simulink model "benchmark_ivan_PIANN"  (R2024b)
settings: Solver=FixedStepAuto  StartTime=0.0  StopTime=14  FixedStep=0.0001  RelTol=1e-5  AbsTol=1e-8  EnableMultiTasking=on
values from neighbouring files (symbols this model uses):
  b1 = csvread('./DAE_ANN/ANN/Biases/30_04_21/lstm_ann_pi_standard_fix_noSo4_rnn_1__100_16_b_3.csv')    [init_PI_ann.m]    (also in init_PI_ann_hier.m = csvread('./DAE_ANN/ANN/Biases/12_05_21/lstm_ann_pi_standard_; init_PI_ann_hier_v2.m = csvread('./DAE_ANN/ANN/Biases/12_05_21/lstm_ann_pi_standard_; init_PI_ann_lab.m = csvread('./DAE_ANN/ANN/Biases/12_05_21/lstm_ann_pi_standard_)
  b2 = csvread('./DAE_ANN/ANN/Biases/30_04_21/lstm_ann_pi_standard_fix_noSo4_rnn_1__100_16_b_3.csv')    [init_PI_ann.m]    (also in init_PI_ann_hier.m = csvread('./DAE_ANN/ANN/Biases/12_05_21/lstm_ann_pi_standard_; init_PI_ann_hier_v2.m = csvread('./DAE_ANN/ANN/Biases/12_05_21/lstm_ann_pi_standard_; init_PI_ann_lab.m = csvread('./DAE_ANN/ANN/Biases/12_05_21/lstm_ann_pi_standard_)
  b_last = csvread('./DAE_ANN/ANN/Biases/12_05_21/lstm_ann_pi_standard_fix_noSo4_last__100_1_b_2.csv')'    [init_PI_ann_hier.m]    (also in init_PI_ann_hier_v2.m; init_PI_ann_lab.m)
  b_out = csvread('./DAE_ANN/ANN/Biases/30_04_21/lstm_ann_pi_standard_fix_noSo4_final__100_16_b_3.csv')    [init_PI_ann.m]    (also in init_PI_ann_hier.m = csvread('./DAE_ANN/ANN/Biases/12_05_21/lstm_ann_pi_standard_; init_PI_ann_hier_v2.m = csvread('./DAE_ANN/ANN/Biases/12_05_21/lstm_ann_pi_standard_; init_PI_ann_lab.m = csvread('./DAE_ANN/ANN/Biases/12_05_21/lstm_ann_pi_standard_)
  ic_sw_Kla = 145*ones(n_sw,1)    [init_PI_ann.m]    (also in init_PI_ann_hier.m; init_PI_ann_hier_v2.m; init_PI_ann_lab.m)
  ic_sw_Snh4 = 6*ones(n_sw,1)    [init_PI_ann.m]    (also in init_PI_ann_hier.m; init_PI_ann_hier_v2.m; init_PI_ann_lab.m)
  ic_sw_Sno4 = 8*ones(n_sw,1)    [init_PI_ann.m]    (also in init_PI_ann_hier.m; init_PI_ann_hier_v2.m; init_PI_ann_lab.m)
  ic_sw_So4 = 3*ones(n_sw,1)    [init_PI_ann.m]    (also in init_PI_ann_hier.m; init_PI_ann_hier_v2.m; init_PI_ann_lab.m)
  ic_sw_So5 = 2*ones(n_sw,1)    [init_PI_ann.m]    (also in init_PI_ann_hier.m; init_PI_ann_hier_v2.m; init_PI_ann_lab.m)
  KLa5_max = 360    [sensorinit.m]
  max_Q4 = 100000    [sensorinit.m]
  max_SNH4 = 20    [sensorinit.m]
  max_SNO2 = 20    [sensorinit.m]
  max_SNO4 = 20    [sensorinit.m]
  max_SO4 = 10    [sensorinit.m]
  max_SO5 = 10    [sensorinit.m]    (also in setup_Prac5.m = 5)
  max_TSS4 = 10000    [sensorinit.m]
  mean_scaler_dir = csvread('./DAE_ANN/ANN/Scalers/30_04_21_lstm_ann_pi_standard_fix_noSo4/mean_scaler_lstm_ann_pi_standard_fix_noSo4.csv')    [init_PI_ann.m]    (also in init_PI_ann_hier.m = csvread('./DAE_ANN/ANN/Scalers/12_05_21_lstm_ann_pi_standard; init_PI_ann_hier_v2.m = csvread('./DAE_ANN/ANN/Scalers/12_05_21_lstm_ann_pi_standard; setup_Prac5.m = [(Q/k)^2, 1.9756, 0.0000, 0]')
  mean_scaler_dir_out = csvread('./DAE_ANN/ANN/Scalers/30_04_21_lstm_ann_pi_standard_fix_noSo4/mean_scaler_lstm_ann_pi_standard_fix_noSo4_out.csv')    [init_PI_ann.m]    (also in init_PI_ann_hier.m = csvread('./DAE_ANN/ANN/Scalers/12_05_21_lstm_ann_pi_standard; init_PI_ann_hier_v2.m = csvread('./DAE_ANN/ANN/Scalers/12_05_21_lstm_ann_pi_standard; setup_Prac5.m = 0)
  min_Q4 = 0    [sensorinit.m]
  min_SNH4 = 0    [sensorinit.m]
  min_SNO2 = 0    [sensorinit.m]
  min_SNO4 = 0    [sensorinit.m]
  min_SO5 = 0    [sensorinit.m]
  min_TSS4 = 0    [sensorinit.m]
  n_layers = 1    [init_PI_ann.m]    (also in init_PI_ann_hier.m; init_PI_ann_hier_v2.m; init_PI_ann_lab.m)
  n_sw = 16    [init_PI_ann.m]    (also in init_PI_ann_hier.m = 1; init_PI_ann_hier_v2.m = 1; init_PI_ann_lab.m = 1)
  n_sw_inverse = 16    [init_PI_ann.m]    (also in init_PI_ann_hier.m = 1; init_PI_ann_hier_v2.m = 1; init_PI_ann_lab.m = 1)
  noiseseed_Q4 = 1    [sensorinit.m]
  noiseseed_SNH4 = 2    [sensorinit.m]
  noiseseed_SNO2 = 2    [sensorinit.m]
  noiseseed_SNO4 = 2    [sensorinit.m]
  noiseseed_SO4 = 2    [sensorinit.m]
  noiseseed_SO5 = 1    [sensorinit.m]
  noiseseed_TSS4 = 1    [sensorinit.m]
  noisesource_Q4 = 1    [sensorinit.m]
  noisesource_SNH4 = 1    [sensorinit.m]
  noisesource_SNO2 = 1    [sensorinit.m]
  noisesource_SNO4 = 1    [sensorinit.m]
  noisesource_SO4 = 1    [sensorinit.m]
  noisesource_SO5 = 1    [sensorinit.m]
  noisesource_TSS4 = 1    [sensorinit.m]
  Qin0 = 18446    [states.mat]
  Qintr = 12141.8126939    [states.mat]
  Qintr_max = 5*Qin0    [sensorinit.m]
  Qintrawstate = 114243.527362    [states.mat]
  Qintrintstate = -116205.765277    [states.mat]
  SETTLERINIT = [12.5979803087 18.2981709885 29.6744598765 68.7829340492 352.293497132 353.981663079 351.499035887 351.323930185 355.679725774 6417.21684783 30 30 ... (80 elements, 1x80)]    [states.mat]
  Sno_mean = 1    [run_bsm1_PIANN_variable.m]
  SO5awstate = 469.399689831    [states.mat]
  SO5intstate = -450.70071346    [states.mat]
  SO5ref = 2    [run_bsm1_PIANN.m]    (also in run_bsm1_PIANN_variable.m)
  So_mean = 2    [run_bsm1_PIANN_variable.m]    (also in setup_Prac5.m = 0.2)
  std_Q4 = 0.025    [sensorinit.m]
  std_scaler_dir = csvread('./DAE_ANN/ANN/Scalers/30_04_21_lstm_ann_pi_standard_fix_noSo4/std_scaler_lstm_ann_pi_standard_fix_noSo4.csv')    [init_PI_ann.m]    (also in init_PI_ann_hier.m = csvread('./DAE_ANN/ANN/Scalers/12_05_21_lstm_ann_pi_standard; init_PI_ann_hier_v2.m = csvread('./DAE_ANN/ANN/Scalers/12_05_21_lstm_ann_pi_standard; setup_Prac5.m = [1, 0.7579, 0.05, 1]')
  std_scaler_dir_out = csvread('./DAE_ANN/ANN/Scalers/30_04_21_lstm_ann_pi_standard_fix_noSo4/std_scaler_lstm_ann_pi_standard_fix_noSo4_out.csv')    [init_PI_ann.m]    (also in init_PI_ann_hier.m = csvread('./DAE_ANN/ANN/Scalers/12_05_21_lstm_ann_pi_standard; init_PI_ann_hier_v2.m = csvread('./DAE_ANN/ANN/Scalers/12_05_21_lstm_ann_pi_standard; setup_Prac5.m = 1)
  std_SNH4 = 0.025    [sensorinit.m]
  std_SNO2 = 0.025    [sensorinit.m]
  std_SO4 = 0.025    [sensorinit.m]
  std_SO5 = 0.025    [sensorinit.m]
  std_TSS4 = 0.025    [sensorinit.m]
  T = 6.5201    [setup_Prac5.m]
  t_init = 7e-3    (= 0.007)    [run_bsm1.m]    (also in run_bsm1_PIANN_variable.m = 0.05)
  T_KLa5 = T90_KLa5/(24*60)/3.89    (= 0.000714081690945)    [sensorinit.m]
  T_Q4 = T90_Q4/(24*60)/3.89    (= 0.000178520422736)    [sensorinit.m]
  t_simulink = 1/96    (= 0.0104166666667)    [run_bsm1.m]    (also in run_bsm1_PIANN.m = -1; run_bsm1_PIANN_variable.m = 0; setup_Prac5.m = 0)
  T_SNH4 = T90_SNH4/(24*60)/11.7724    (= 0.000589891988417)    [sensorinit.m]
  T_SNO2 = T90_SNO2/(24*60)/11.7724    (= 0.000589891988417)    [sensorinit.m]
  T_SNO4 = T90_SNO4/(24*60)/11.7724    (= 0.000589891988417)    [sensorinit.m]
  T_SO5 = T90_SO5/(24*60)/3.89    (= 0.000178520422736)    [sensorinit.m]
  T_TSS4 = T90_TSS4/(24*60)/3.89    (= 0.000178520422736)    [sensorinit.m]
  t_zero_order = -1    [run_bsm1_PIANN.m]    (also in run_bsm1_PIANN_variable.m)
  u1 = csvread('./DAE_ANN/ANN/Weights/30_04_21/lstm_ann_pi_standard_fix_noSo4_rnn_1__100_16_U_3.csv')    [init_PI_ann.m]    (also in init_PI_ann_hier.m = csvread('./DAE_ANN/ANN/Weights/12_05_21/lstm_ann_pi_standard; init_PI_ann_hier_v2.m = csvread('./DAE_ANN/ANN/Weights/12_05_21/lstm_ann_pi_standard)
  u2 = csvread('./DAE_ANN/ANN/Weights/30_04_21/lstm_ann_pi_standard_fix_noSo4_rnn_1__100_16_U_3.csv')    [init_PI_ann.m]    (also in init_PI_ann_hier.m = csvread('./DAE_ANN/ANN/Weights/12_05_21/lstm_ann_pi_standard; init_PI_ann_hier_v2.m = csvread('./DAE_ANN/ANN/Weights/12_05_21/lstm_ann_pi_standard)
  useideal_KLa5 = 0    [run_bsm1.m]    (also in run_bsm1_PIANN.m = 1; run_bsm1_PIANN_variable.m = 1; sensorinit.m)
  useideal_Q4 = 1    [run_bsm1_PIANN.m]    (also in run_bsm1_PIANN_variable.m; sensorinit.m = 0)
  useideal_SNH4 = 0    [run_bsm1.m]    (also in run_bsm1_PIANN.m = 1; run_bsm1_PIANN_variable.m = 1; sensorinit.m)
  useideal_SNO2 = 1    [run_bsm1_PIANN.m]    (also in run_bsm1_PIANN_variable.m; sensorinit.m = 0)
  useideal_SNO4 = 0    [run_bsm1.m]    (also in run_bsm1_PIANN.m = 1; run_bsm1_PIANN_variable.m = 1; sensorinit.m)
  useideal_SO4 = 0    [run_bsm1.m]    (also in run_bsm1_PIANN.m = 1; run_bsm1_PIANN_variable.m = 1; sensorinit.m)
  useideal_SO5 = 0    [run_bsm1.m]    (also in run_bsm1_PIANN.m = 1; run_bsm1_PIANN_variable.m = 1; sensorinit.m)
  useideal_TSS4 = 1    [run_bsm1_PIANN.m]    (also in run_bsm1_PIANN_variable.m; sensorinit.m = 0)
  usenoise_Q4 = 0    [run_bsm1_PIANN.m]    (also in run_bsm1_PIANN_variable.m; sensorinit.m = 1)
  usenoise_SNH4 = 1    [run_bsm1.m]    (also in run_bsm1_PIANN.m = 0; run_bsm1_PIANN_variable.m = 0; sensorinit.m)
  usenoise_SNO2 = 0    [run_bsm1_PIANN.m]    (also in run_bsm1_PIANN_variable.m; sensorinit.m = 1)
  usenoise_SNO4 = 1    [run_bsm1.m]    (also in run_bsm1_PIANN.m = 0; run_bsm1_PIANN_variable.m = 0; sensorinit.m)
  usenoise_SO4 = 1    [run_bsm1.m]    (also in run_bsm1_PIANN.m = 0; run_bsm1_PIANN_variable.m = 0; sensorinit.m)
  usenoise_SO5 = 1    [run_bsm1.m]    (also in run_bsm1_PIANN.m = 0; run_bsm1_PIANN_variable.m = 0; sensorinit.m)
  usenoise_TSS4 = 0    [run_bsm1_PIANN.m]    (also in run_bsm1_PIANN_variable.m; sensorinit.m = 1)
  w1 = csvread('./DAE_ANN/ANN/Weights/30_04_21/lstm_ann_pi_standard_fix_noSo4_rnn_1__100_16_W_3.csv')    [init_PI_ann.m]    (also in init_PI_ann_hier.m = csvread('./DAE_ANN/ANN/Weights/12_05_21/lstm_ann_pi_standard; init_PI_ann_hier_v2.m = csvread('./DAE_ANN/ANN/Weights/12_05_21/lstm_ann_pi_standard; init_PI_ann_lab.m = csvread('./DAE_ANN/ANN/Weights/12_05_21/lstm_ann_pi_standard)
  w2 = csvread('./DAE_ANN/ANN/Weights/30_04_21/lstm_ann_pi_standard_fix_noSo4_rnn_1__100_16_W_3.csv')    [init_PI_ann.m]    (also in init_PI_ann_hier.m = csvread('./DAE_ANN/ANN/Weights/12_05_21/lstm_ann_pi_standard; init_PI_ann_hier_v2.m = csvread('./DAE_ANN/ANN/Weights/12_05_21/lstm_ann_pi_standard; init_PI_ann_lab.m = csvread('./DAE_ANN/ANN/Weights/12_05_21/lstm_ann_pi_standard)
  w_last = csvread('./DAE_ANN/ANN/Weights/12_05_21/lstm_ann_pi_standard_fix_noSo4_last__100_1_W_2.csv')    [init_PI_ann_hier.m]    (also in init_PI_ann_hier_v2.m; init_PI_ann_lab.m)
  w_out = csvread('./DAE_ANN/ANN/Weights/30_04_21/lstm_ann_pi_standard_fix_noSo4_final__100_16_W_3.csv')    [init_PI_ann.m]    (also in init_PI_ann_hier.m = csvread('./DAE_ANN/ANN/Weights/12_05_21/lstm_ann_pi_standard; init_PI_ann_hier_v2.m = csvread('./DAE_ANN/ANN/Weights/12_05_21/lstm_ann_pi_standard; init_PI_ann_lab.m = csvread('./DAE_ANN/ANN/Weights/12_05_21/lstm_ann_pi_standard)
  XINIT1 = [30 3.2250440682 1132.84750814 98.0848162551 2520.32093658 147.34360098 454.498440184 0.006943357113 3.54207658602 12.0720627837 1.35151294762 6.05742445882 ... (15 elements, 1x15)]    [states.mat]
  XINIT2 = [30 1.63865407136 1124.24951453 88.653599068 2501.35826654 146.001740625 452.094465666 5.17099136584e-05 1.14245691502 13.0383387996 0.796493225193 5.70045637375 ... (15 elements, 1x15)]    [states.mat]
  XINIT3 = [30 1.20592174915 1120.58961418 67.1871738861 2499.94635325 146.547839977 452.007772249 1.74081325353 6.26492922945 8.40116301472 0.827753486834 4.51387309735 ... (15 elements, 1x15)]    [states.mat]
  XINIT4 = [30 0.96656120797 1121.66055561 52.7833355811 2504.32671079 147.644975737 453.890499756 2.40137566232 11.073804945 3.99279026202 0.746788866766 3.70339113264 ... (15 elements, 1x15)]    [states.mat]
  XINIT5 = [30 0.803395489358 1124.12455116 43.2595495328 2508.23031357 148.499403125 456.322790044 2.11978031988 14.1356901459 1.15379834533 0.659650038761 3.15951382084 ... (15 elements, 1x15)]    [states.mat]
  XINITDELAY = [1466770.04249 1266021.87556 55799754.9774 5815431.95778 123179806.598 7263098.80912 22318785.5012 62039.7687555 416609.519268 588047.303413 143684.636473 343270.852984 ... (15 elements, 1x15)]    [states.mat]
undefined symbols (not defined in the file or in its folder): b_bottle, b_decoder_1, b_decoder_2, b_encoder_1, b_encoder_2, b_final, b_out_dae, carb1, carb2, carb3, carb4, carb5, DIM, Kfeedforward, KLa1, KLa2, KLa3, KLa4, KLa5offset, KQintr, KSO5, LAYER, magnitude, mean_scaler_dae, mean_scaler_dae_out, MODELTYPE, PAR1, PAR2, PAR3, PAR4, PAR5, Qffref, Qintroffset, QintrT, SETTLERPAR, SNO2ref, SOSAT1, SOSAT2, SOSAT3, SOSAT4, SOSAT5, std_scaler_dae, std_scaler_dae_out, TiQintr, TiSO5, TtQintr, TtSO5, u_decoder_1, u_decoder_2, u_encoder_1, u_encoder_2, useantiwindupQintr, useantiwindupSO5, VOL1, VOL2, VOL3, VOL4, VOL5, w_bottle, w_decoder_1 ... (+5)
libraries: dspindex x33
(part 1 of 4)
settings Model: Creator=ielulf  LastModifiedBy=1630327
settings SolverCC: AutoScaleAbsTol=off  ConcurrentTasks=on  AlgebraicLoopSolver=LineSearch  PositivePriorityOrder=on  AutoInsertRateTranBlk=on
settings DataIOCC: SaveFormat=StructureWithTime  SignalLoggingSaveFormat=ModelDataLogs  SaveOutput=off  ReturnWorkspaceOutputs=off  TimeSaveName=t  SignalLoggingName=sigsOut  OutputOption=SpecifiedOutputTimes  OutputTimes=[0:(1/96):14]
settings OptimizationCC: BlockReduction=off  BooleanDataType=off  DefaultParameterBehavior=Inlined  OptimizeBlockIOStorage=off  InitFltsAndDblsToZero=on
settings DebuggingCC: AlgebraicLoopMsg=none  SaveWithParameterizedLinksMsg=none  UnderspecifiedInitializationDetection=Classic  MergeDetectMultiDrivingBlocksExec=none  SignalResolutionControl=TryResolveAllWithWarning  InheritedTsInSrcMsg=none  TasksWithSamePriorityMsg=none  FcnCallInpInsideContextMsg=warning  UnconnectedInputMsg=warning  UnconnectedLineMsg=warning  SFUnexpectedBacktrackingDiag=warning  SFNoUnconditionalDefaultTransitionDiag=warning  SFExecutionAtInitializationDiag=none  ArithmeticOperatorsInVariantConditions=warning
settings HardwareCC: ProdBitPerLong=64  ProdLongLongMode=on  ProdHWDeviceType=Intel->x86-64 (Linux 64)  TargetBitPerPointer=64  TargetBitPerSizeT=64  TargetBitPerPtrDiffT=64  TargetLongLongMode=on  TargetIntDivRoundTo=Zero  TargetEndianess=LittleEndian  TargetWordSize=64  TargetHWDeviceType=MATLAB Host
settings ModelReferenceCC: EnableRefExpFcnMdlSchedulingChecks=on  PropagateSignalLabelsOutOfModel=off
settings SFSimCC: SimUseLocalCustomCode=off  CustomCodeUndefinedFunction=UseInterfaceOnly
settings RTWCC: Description=Speedgoat Real-Time Target Machine  SystemTargetFile=speedgoat.tlc  TemplateMakefile=slrealtime_default_tmf  RTWUseLocalCustomCode=off  Toolchain=Simulink Real-Time Toolchain  BuildConfiguration=Faster Runs  CodeExecutionProfiling=on  TargetLang=C++  GPUComputeCapability=3.5  DLArmComputeVersion=19.05
settings CodeAppCC: StateflowObjectComments=on
settings SimulinkRealTimeTargetCC: InstructionSetFMA=off  LogToMDFFile=off
settings ConfigComp: CovMetricSettings=dw  CovSaveCumulativeToWorkspaceVar=on  CovSaveSingleToWorkspaceVar=on  CovExternalEMLEnable=off

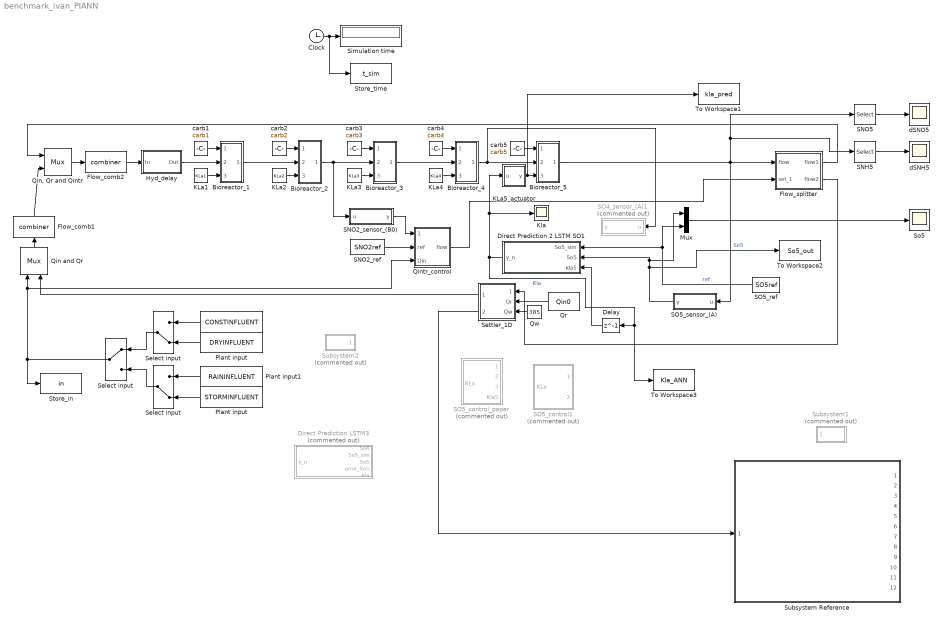
== system benchmark_ivan_PIANN ==
  " " : FromWorkspace  VariableName=CONSTINFLUENT  SampleTime=-1  ZeroCross=off  OutputAfterFinalValue=Holding final value
  " Select input" : ManualSwitch
  Bioreactor_1 : Subsystem
  Bioreactor_2 : Subsystem
  Bioreactor_3 : Subsystem
  Bioreactor_4 : Subsystem
  Bioreactor_5 : Subsystem
  Clock : Clock
  Delay : Delay  DelayLength=1  InitialCondition=0
  Direct Prediction 2 LSTM SO1 : Subsystem
  Direct Prediction LSTM3 : Subsystem  Commented=on
  Flow_comb1 : S-Function  FunctionName=combiner  SFunctionDeploymentMode=off  EnableBusSupport=off
  Flow_comb2 : S-Function  FunctionName=combiner  SFunctionDeploymentMode=off  EnableBusSupport=off
  Flow_splitter : Subsystem
  Hyd_delay : Subsystem
  KLa1 : Constant  Value=KLa1
  KLa2 : Constant  Value=KLa2
  KLa3 : Constant  Value=KLa3
  KLa4 : Constant  Value=KLa4
  KLa5_actuator : Subsystem
  Kla : Scope
  Mux : Mux  Inputs=2
  Plant input : FromWorkspace  VariableName=DRYINFLUENT  SampleTime=-1  ZeroCross=off  OutputAfterFinalValue=Holding final value
  "Plant input " : FromWorkspace  VariableName=STORMINFLUENT  SampleTime=-1  ZeroCross=off  OutputAfterFinalValue=Holding final value
  Plant input1 : FromWorkspace  VariableName=RAININFLUENT  SampleTime=-1  ZeroCross=off  OutputAfterFinalValue=Holding final value
  Qin and Qr : Mux  Inputs=2
  "Qin, Qr and Qintr" : Mux  Inputs=2
  Qintr_control : Subsystem
  Qr : Constant  Value=Qin0
  Qw : Constant  Value=385
  SNH5 : Selector  InputPortWidth=15  IndexOptions=Index vector (dialog)  Indices=[9]  OutputSizes=1
  SNO2_ref : Constant  Value=SNO2ref
  SNO2_sensor_(B0) : Subsystem
  SNO5 : Selector  InputPortWidth=15  IndexOptions=Index vector (dialog)  Indices=[9]  OutputSizes=1
  SO4_sensor_(A)1 : Subsystem  Commented=on
  SO5_control1 : Subsystem  Commented=on
  SO5_control_paper : Subsystem  Commented=on
  SO5_ref : Constant  Value=SO5ref
  SO5_sensor_(A) : Subsystem
  Select input : ManualSwitch  CurrentSetting=0
  "Select input " : ManualSwitch  CurrentSetting=0
  Settler_1D : Subsystem
  Simulation time : Display
  So5 : Scope
  Store_in : ToWorkspace  VariableName=in
  Store_time : ToWorkspace  VariableName=t_sim
  Subsystem Reference : Subsystem  ReferencedSubsystem=Plot_Performance
  Subsystem1 : Subsystem  Commented=on
  Subsystem2 : Subsystem  Commented=on
  To Workspace1 : ToWorkspace  VariableName=kla_pred  SampleTime=-1
  To Workspace2 : ToWorkspace  VariableName=So5_out  SampleTime=-1
  To Workspace3 : ToWorkspace  VariableName=Kla_ANN  SampleTime=-1
  carb1 : Constant  Value=carb1
  carb2 : Constant  Value=carb2
  carb3 : Constant  Value=carb3
  carb4 : Constant  Value=carb4
  carb5 : Constant  Value=carb5
  dSNH5 : Scope
  dSNO5 : Scope
  wires:
  Qin and Qr/1 -> Flow_comb1/1
  Flow_comb1/1 -> "Qin, Qr and Qintr"/2
  "Qin, Qr and Qintr"/1 -> Flow_comb2/1
  Flow_splitter/1(flow1) -> "Qin, Qr and Qintr"/1
  Settler_1D/1(output) -> Qin and Qr/2
  Qw/1 -> Settler_1D/3(Qw)
  Flow_splitter/2(flow2) -> Settler_1D/1(feed)
  Qr/1 -> Settler_1D/2(Qr)
  Flow_comb2/1 -> Hyd_delay/1(In)
  Clock/1 -> Store_time/1, Simulation time/1
  Plant input/1 -> Select input/2
  " "/1 -> Select input/1
  Hyd_delay/1(Out) -> Bioreactor_1/2(in)
  carb1/1 -> Bioreactor_1/1(carb)
  KLa1/1 -> Bioreactor_1/3(KLa)
  Bioreactor_1/1(out) -> Bioreactor_2/2(in)
  KLa2/1 -> Bioreactor_2/3(KLa)
  carb2/1 -> Bioreactor_2/1(carb)
  Bioreactor_2/1(out) -> Bioreactor_3/2(in), SNO2_sensor_(B0)/1(u)
  KLa3/1 -> Bioreactor_3/3(KLa)
  carb3/1 -> Bioreactor_3/1(carb)
  Bioreactor_3/1(out) -> Bioreactor_4/2(in)
  KLa4/1 -> Bioreactor_4/3(KLa)
  carb4/1 -> Bioreactor_4/1(carb)
  carb5/1 -> Bioreactor_5/1(carb)
  Plant input1/1 -> "Select input "/1
  "Plant input "/1 -> "Select input "/2
  Select input/1 -> " Select input"/1
  "Select input "/1 -> " Select input"/2
  " Select input"/1 -> Store_in/1, Qin and Qr/1, Qintr_control/3(Qin)
  SNO2_ref/1 -> Qintr_control/2(ref)
  SNO2_sensor_(B0)/1(y) -> Qintr_control/1(meas)
  Qintr_control/1(flow) -> Flow_splitter/2(set_1)
  KLa5_actuator/1(y) -> To Workspace1/1, Bioreactor_5/3(KLa)
  Direct Prediction 2 LSTM SO1/1(y_n) -> KLa5_actuator/1(u), Kla/1, To Workspace3/1, Delay/1  "Kla"
  Bioreactor_5/1(out) -> SNH5/1, SNO5/1, Flow_splitter/1(flow), SO5_sensor_(A)/1(u)
  Mux/1 -> So5/1
  Bioreactor_4/1(out) -> Bioreactor_5/2(in), SO4_sensor_(A)1/1(u)
  SO5_ref/1 -> Direct Prediction 2 LSTM SO1/1(So5_sim), Mux/2  "ref"
  SO5_sensor_(A)/1(y) -> To Workspace2/1, Direct Prediction 2 LSTM SO1/2(So5), Mux/1  "So5"
  Delay/1 -> Direct Prediction 2 LSTM SO1/3(kla5)
  SNO5/1 -> dSNO5/1
  SNH5/1 -> dSNH5/1
  Settler_1D/2(Settler) -> Subsystem Reference/1

== system benchmark_ivan_PIANN/Bioreactor_1 ==
  carb : Inport
  in : Inport  Port=2
  KLa : Inport  Port=3
  Bioreactor_1 : S-Function  FunctionName=asm1  Parameters=XINIT1,PAR1,VOL1,SOSAT1  SFunctionDeploymentMode=off  EnableBusSupport=off
  Carboncombiner : Subsystem
  Store_KLa1 : ToWorkspace  VariableName=kla1in
  Store_carb1 : ToWorkspace  VariableName=carbon1in
  Store_reac1 : ToWorkspace  VariableName=reac1  SampleTime=-1
  add KLa : Mux  Inputs=2
  out : Outport  VectorParamsAs1DForOutWhenUnconnected=off
  wires:
  add KLa/1 -> Bioreactor_1/1
  Bioreactor_1/1 -> out/1, Store_reac1/1
  Carboncombiner/1(Output) -> add KLa/1
  carb/1 -> Store_carb1/1, Carboncombiner/1(C_flow)
  in/1 -> Carboncombiner/2(Input)
  KLa/1 -> add KLa/2, Store_KLa1/1

== system benchmark_ivan_PIANN/Bioreactor_2 ==
  carb : Inport
  in : Inport  Port=2
  KLa : Inport  Port=3
  Bioreactor_2 : S-Function  FunctionName=asm1  Parameters=XINIT2,PAR2,VOL2,SOSAT2  SFunctionDeploymentMode=off  EnableBusSupport=off
  Carboncombiner : Subsystem
  Store_KLa2 : ToWorkspace  VariableName=kla2in
  Store_carb2 : ToWorkspace  VariableName=carbon2in
  Store_reac2 : ToWorkspace  VariableName=reac2  SampleTime=-1
  add KLa : Mux  Inputs=2
  out : Outport  VectorParamsAs1DForOutWhenUnconnected=off
  wires:
  Bioreactor_2/1 -> out/1, Store_reac2/1
  add KLa/1 -> Bioreactor_2/1
  Carboncombiner/1(Output) -> add KLa/1
  carb/1 -> Carboncombiner/1(C_flow), Store_carb2/1
  in/1 -> Carboncombiner/2(Input)
  KLa/1 -> add KLa/2, Store_KLa2/1

== system benchmark_ivan_PIANN/Bioreactor_3 ==
  carb : Inport
  in : Inport  Port=2
  KLa : Inport  Port=3
  Bioreactor_3 : S-Function  FunctionName=asm1  Parameters=XINIT3,PAR3,VOL3,SOSAT3  SFunctionDeploymentMode=off  EnableBusSupport=off
  Carboncombiner : Subsystem
  Store_KLa : ToWorkspace  VariableName=kla3in
  Store_carb3 : ToWorkspace  VariableName=carbon3in
  Store_reac1 : ToWorkspace  VariableName=reac3  SampleTime=-1
  add KLa : Mux  Inputs=2
  out : Outport  VectorParamsAs1DForOutWhenUnconnected=off
  wires:
  Bioreactor_3/1 -> out/1, Store_reac1/1
  add KLa/1 -> Bioreactor_3/1
  Carboncombiner/1(Output) -> add KLa/1
  carb/1 -> Carboncombiner/1(C_flow), Store_carb3/1
  in/1 -> Carboncombiner/2(Input)
  KLa/1 -> add KLa/2, Store_KLa/1

== system benchmark_ivan_PIANN/Bioreactor_4 ==
  carb : Inport
  in : Inport  Port=2
  KLa : Inport  Port=3
  Bioreactor_4 : S-Function  FunctionName=asm1  Parameters=XINIT4,PAR4,VOL4,SOSAT4  SFunctionDeploymentMode=off  EnableBusSupport=off
  Carboncombiner : Subsystem
  Store_KLa4 : ToWorkspace  VariableName=kla4in
  Store_carb4 : ToWorkspace  VariableName=carbon4in
  Store_reac4 : ToWorkspace  VariableName=reac4  SampleTime=-1
  add KLa : Mux  Inputs=2
  out : Outport  VectorParamsAs1DForOutWhenUnconnected=off
  wires:
  Bioreactor_4/1 -> out/1, Store_reac4/1
  add KLa/1 -> Bioreactor_4/1
  Carboncombiner/1(Output) -> add KLa/1
  carb/1 -> Carboncombiner/1(C_flow), Store_carb4/1
  in/1 -> Carboncombiner/2(Input)
  KLa/1 -> add KLa/2, Store_KLa4/1

== system benchmark_ivan_PIANN/Bioreactor_5 ==
  carb : Inport
  in : Inport  Port=2
  KLa : Inport  Port=3
  Bioreactor_5 : S-Function  FunctionName=asm1  Parameters=XINIT5,PAR5,VOL5,SOSAT5  SFunctionDeploymentMode=off  EnableBusSupport=off
  Carboncombiner : Subsystem
  Store_KLa5 : ToWorkspace  VariableName=kla5in
  Store_carb5 : ToWorkspace  VariableName=carbon5in
  Store_reac5 : ToWorkspace  VariableName=reac5  SampleTime=-1
  add KLa : Mux  Inputs=2
  out : Outport  VectorParamsAs1DForOutWhenUnconnected=off
  wires:
  Bioreactor_5/1 -> out/1, Store_reac5/1
  add KLa/1 -> Bioreactor_5/1
  Carboncombiner/1(Output) -> add KLa/1
  carb/1 -> Carboncombiner/1(C_flow), Store_carb5/1
  in/1 -> Carboncombiner/2(Input)
  KLa/1 -> add KLa/2, Store_KLa5/1

== system benchmark_ivan_PIANN/Direct Prediction 2 LSTM SO1 ==
  So5_sim : Inport
  So5 : Inport  Port=2
  kla5 : Inport  Port=3
  Add : Sum  Inputs=+-
  Data Preprocesing Direct : Subsystem
  Data Preprocessing Direct1 : Subsystem
  Direct ANN1 : Subsystem
  IAE_ISE : Subsystem
  Memory : Memory
  Saturation : Saturate  UpperLimit=360  LowerLimit=0
  Sliding Window : Subsystem
  y_n : Outport  VectorParamsAs1DForOutWhenUnconnected=off
  wires:
  kla5/1 -> Sliding Window/4(kla)
  Add/1 -> Sliding Window/3(errorSo5), IAE_ISE/1(In1)
  So5/1 -> Sliding Window/2(So5out), Add/1
  So5_sim/1 -> Sliding Window/1(So5sim), Add/2
  Sliding Window/1(Out1) -> Data Preprocesing Direct/1(u_n)
  Data Preprocessing Direct1/1(Out1) -> Saturation/1
  Direct ANN1/1(y_n) -> Data Preprocessing Direct1/1(y_n)
  Data Preprocesing Direct/1(Out1) -> Direct ANN1/1(x_norm)
  Saturation/1 -> Memory/1
  Memory/1 -> y_n/1

== system benchmark_ivan_PIANN/Direct Prediction LSTM3 ==
  So4 : Inport
  So5_sim : Inport  Port=2
  So5 : Inport  Port=3
  error_So5 : Inport  Port=4
  kla : Inport  Port=5
  Data Preprocesing Direct : Subsystem
  Data Preprocessing Direct1 : Subsystem
  Direct ANN : Subsystem
  Saturation : Saturate  UpperLimit=360  LowerLimit=0
  Sliding Window : Subsystem
  y_n : Outport  VectorParamsAs1DForOutWhenUnconnected=off
  wires:
  Data Preprocesing Direct/1(Out1) -> Direct ANN/1(x_norm)
  Direct ANN/1(y_n) -> Data Preprocessing Direct1/1(y_n)
  Data Preprocessing Direct1/1(Out1) -> Saturation/1
  Sliding Window/1(Out1) -> Data Preprocesing Direct/1(u_n)
  Saturation/1 -> y_n/1
  So5_sim/1 -> Sliding Window/2(So5sim)
  So5/1 -> Sliding Window/3(So5out)
  error_So5/1 -> Sliding Window/4(errorSo5)
  So4/1 -> Sliding Window/1(So4)
  kla/1 -> Sliding Window/5(kla)

== system benchmark_ivan_PIANN/Flow_splitter ==
  flow : Inport
  set_1 : Inport  Port=2
  Mux : Mux  Inputs=2
  Mux1 : Mux  Inputs=2
  Selector : Selector  InputPortWidth=15  IndexOptions=Index vector (dialog)  Indices=[15]  OutputSizes=1
  Selector1 : Selector  InputPortWidth=15  IndexOptions=Index vector (dialog)  Indices=[1 2 3 4 5 6 7 8 9 10 11 12 13 14]  OutputSizes=1
  Store_rec : ToWorkspace  VariableName=rec  SampleTime=-1
  Sum : Sum  Inputs=-+  InputSameDT=on  SaturateOnIntegerOverflow=on  OutDataTypeStr=Inherit: Same as first input
  flow1 : Outport  VectorParamsAs1DForOutWhenUnconnected=off
  flow2 : Outport  Port=2  VectorParamsAs1DForOutWhenUnconnected=off
  wires:
  flow/1 -> Selector1/1, Selector/1
  Mux/1 -> flow1/1, Store_rec/1
  Mux1/1 -> flow2/1
  set_1/1 -> Mux/2, Sum/1
  Selector/1 -> Sum/2
  Sum/1 -> Mux1/2
  Selector1/1 -> Mux/1, Mux1/1

== system benchmark_ivan_PIANN/Hyd_delay ==
  In : Inport
  Demux : Demux  Outputs=[14,1]
      settings: DisplayOption=none
  Hyd_delay : S-Function  FunctionName=hyddelayv3  Parameters=XINITDELAY,PAR1,T  SFunctionDeploymentMode=off  EnableBusSupport=off
  Mux : Mux  Inputs=2
  Product : Product  SaturateOnIntegerOverflow=on  OutDataTypeStr=Inherit: Same as first input
  Store_ASinput : ToWorkspace  VariableName=ASinput  SampleTime=-1
  Out : Outport  VectorParamsAs1DForOutWhenUnconnected=off
  wires:
  In/1 -> Hyd_delay/1
  Hyd_delay/1 -> Out/1, Demux/1
  Demux/1 -> Product/1
  Demux/2 -> Product/2, Mux/2
  Product/1 -> Mux/1
  Mux/1 -> Store_ASinput/1

== system benchmark_ivan_PIANN/KLa5_actuator ==
  u : Inport
  Constant2 : Constant  Value=useideal_KLa5
  KLa5_actuator : TransferFcn  Denominator=[ T_KLa5*T_KLa5, 2*T_KLa5, 1]
  Switch1 : Switch  Threshold=0.5  SaturateOnIntegerOverflow=off  InputSameDT=off
  y : Outport  VectorParamsAs1DForOutWhenUnconnected=off
  wires:
  u/1 -> KLa5_actuator/1, Switch1/1
  Switch1/1 -> y/1
  KLa5_actuator/1 -> Switch1/3
  Constant2/1 -> Switch1/2

== system benchmark_ivan_PIANN/Qintr_control ==
  meas : Inport
  ref : Inport  Port=2
  Qin : Inport  Port=3
  Selector : Selector  InputPortWidth=15  IndexOptions=Index vector (dialog)  Indices=[15]  OutputSizes=1
  Sum : Sum  Inputs=-+  InputSameDT=on  SaturateOnIntegerOverflow=on  OutDataTypeStr=Inherit: Same as first input
  cont_PI2 : Subsystem
  flow : Outport  VectorParamsAs1DForOutWhenUnconnected=off
  wires:
  meas/1 -> Sum/1
  Sum/1 -> cont_PI2/1(Error)
  cont_PI2/1(Out) -> flow/1
  Qin/1 -> Selector/1
  ref/1 -> Sum/2, cont_PI2/2(SNOref)
  Selector/1 -> cont_PI2/3(Qin)

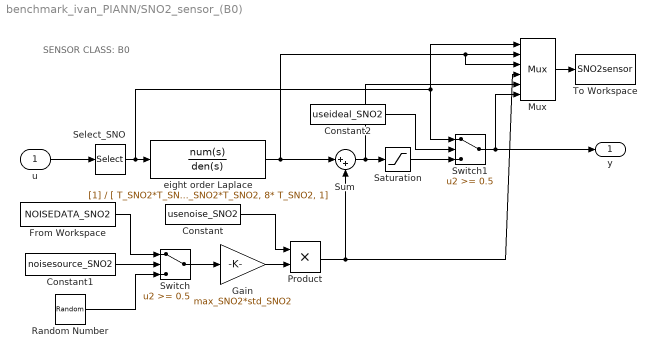
== system benchmark_ivan_PIANN/SNO2_sensor_(B0) ==
  note: SENSOR CLASS: B0
  u : Inport
  Constant : Constant  Value=usenoise_SNO2
  Constant1 : Constant  Value=noisesource_SNO2
  Constant2 : Constant  Value=useideal_SNO2
  From Workspace : FromWorkspace  VariableName=NOISEDATA_SNO2  ZeroCross=off
  Gain : Gain  Gain=max_SNO2*std_SNO2  SaturateOnIntegerOverflow=on  OutDataTypeStr=Inherit: Same as input  ParamDataTypeStr=Inherit: Same as input
  Mux : Mux  Inputs=6
  Product : Product  InputSameDT=on  SaturateOnIntegerOverflow=on  OutDataTypeStr=Inherit: Same as first input
  Random Number : RandomNumber  Seed=noiseseed_SNO2  SampleTime=1/10000
  Saturation : Saturate  UpperLimit=max_SNO2  LowerLimit=min_SNO2
  Select_SNO : Selector  InputPortWidth=15  IndexOptions=Index vector (dialog)  Indices=[9]  OutputSizes=1
  Sum : Sum  Inputs=|++  InputSameDT=on  SaturateOnIntegerOverflow=on  OutDataTypeStr=Inherit: Same as first input
  Switch : Switch  Threshold=0.5  SaturateOnIntegerOverflow=off  InputSameDT=off
  Switch1 : Switch  Threshold=0.5  SaturateOnIntegerOverflow=off  InputSameDT=off
  To Workspace : ToWorkspace  VariableName=SNO2sensor  SampleTime=-1
  eight order Laplace : TransferFcn  Denominator=[ T_SNO2*T_SNO2*T_SNO2*T_SNO2*T_SNO2*T_SNO2*T_SNO2*T_SNO2, 8*T_SNO2*T_SNO2*T_SNO2*T_SNO2*T_SNO2*T_SNO2*T_SNO2, 28*T_SNO2*T_SNO2*T_SNO2*T_SNO2*T_SNO2*T_SNO2, 56*T_SNO2*T_SNO2*T_SNO2*T_SNO2*T_SNO2, 70*T_SNO2*T_SNO2*T_SNO2*T_SNO2, 56*T_SNO2*T_SNO2*T_SNO2, 28*T_SNO2*T_SNO2, 8* T_SNO2, 1]
  y : Outport  VectorParamsAs1DForOutWhenUnconnected=off
  wires:
  Mux/1 -> To Workspace/1
  Constant2/1 -> Switch1/2
  Switch1/1 -> Mux/6, y/1
  Saturation/1 -> Switch1/3
  Random Number/1 -> Switch/3
  Constant1/1 -> Switch/2
  From Workspace/1 -> Switch/1
  Constant/1 -> Product/1
  Switch/1 -> Gain/1
  Gain/1 -> Product/2
  Select_SNO/1 -> Mux/1, Switch1/1, eight order Laplace/1
  u/1 -> Select_SNO/1
  Product/1 -> Mux/4, Sum/2
  eight order Laplace/1 -> Mux/3, Mux/2, Sum/1
  Sum/1 -> Mux/5, Saturation/1

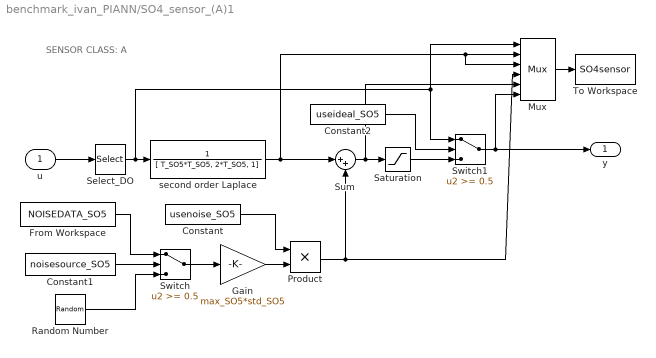
== system benchmark_ivan_PIANN/SO4_sensor_(A)1 ==
  note: SENSOR CLASS: A
  u : Inport
  Constant : Constant  Value=usenoise_SO5
  Constant1 : Constant  Value=noisesource_SO5
  Constant2 : Constant  Value=useideal_SO5
  From Workspace : FromWorkspace  VariableName=NOISEDATA_SO5  ZeroCross=off
  Gain : Gain  Gain=max_SO5*std_SO5  SaturateOnIntegerOverflow=on  OutDataTypeStr=Inherit: Same as input  ParamDataTypeStr=Inherit: Same as input
  Mux : Mux  Inputs=6
  Product : Product  InputSameDT=on  SaturateOnIntegerOverflow=on  OutDataTypeStr=Inherit: Same as first input
  Random Number : RandomNumber  Seed=noiseseed_SO5  SampleTime=1/1440
  Saturation : Saturate  UpperLimit=max_SO5  LowerLimit=min_SO5
  Select_DO : Selector  InputPortWidth=15  IndexOptions=Index vector (dialog)  Indices=[8]  OutputSizes=1
  Sum : Sum  Inputs=|++  InputSameDT=on  SaturateOnIntegerOverflow=on  OutDataTypeStr=Inherit: Same as first input
  Switch : Switch  Threshold=0.5  SaturateOnIntegerOverflow=off  InputSameDT=off
  Switch1 : Switch  Threshold=0.5  SaturateOnIntegerOverflow=off  InputSameDT=off
  To Workspace : ToWorkspace  VariableName=SO4sensor  SampleTime=-1
  second order Laplace : TransferFcn  Denominator=[ T_SO5*T_SO5, 2*T_SO5, 1]
  y : Outport  VectorParamsAs1DForOutWhenUnconnected=off
  wires:
  Mux/1 -> To Workspace/1
  Constant2/1 -> Switch1/2
  Switch1/1 -> Mux/6, y/1
  Saturation/1 -> Switch1/3
  Random Number/1 -> Switch/3
  Constant1/1 -> Switch/2
  From Workspace/1 -> Switch/1
  Constant/1 -> Product/1
  Switch/1 -> Gain/1
  Gain/1 -> Product/2
  Select_DO/1 -> Mux/1, Switch1/1, second order Laplace/1
  u/1 -> Select_DO/1
  Product/1 -> Mux/4, Sum/2
  second order Laplace/1 -> Mux/3, Mux/2, Sum/1
  Sum/1 -> Mux/5, Saturation/1

== system benchmark_ivan_PIANN/SO5_control1 ==
  O2_ref : Inport
  O2_meas : Inport  Port=2
  Abs1 : Abs  SaturateOnIntegerOverflow=off
  Clock : Clock
  Constant : Constant  Value=0
  Filter_Prediction1 : Subsystem  Commented=on
  Integrator2 : Integrator
  Integrator3 : Integrator
  Math Function1 : Math  Operator=magnitude^2  SignedPower=on
  Sum : Sum  Inputs=+-  InputSameDT=on  SaturateOnIntegerOverflow=on  OutDataTypeStr=Inherit: Same as first input
  Switch : Switch  Criteria=u2 > Threshold  Threshold=7  SaturateOnIntegerOverflow=off  InputSameDT=off
  To Workspace1 : ToWorkspace  VariableName=ISE_2  SampleTime=1/96
  To Workspace2 : ToWorkspace  VariableName=IAE_2  SampleTime=1/96
  cont_PI : Subsystem
  KLa : Outport  VectorParamsAs1DForOutWhenUnconnected=off
  wires:
  cont_PI/1(Out) -> KLa/1
  Sum/1 -> Switch/1, cont_PI/1(In)
  Math Function1/1 -> Integrator2/1
  Integrator2/1 -> To Workspace1/1
  Integrator3/1 -> To Workspace2/1
  Abs1/1 -> Integrator3/1
  Clock/1 -> Switch/2
  Switch/1 -> Abs1/1, Math Function1/1
  Constant/1 -> Switch/3
  O2_ref/1 -> Sum/1
  O2_meas/1 -> Sum/2

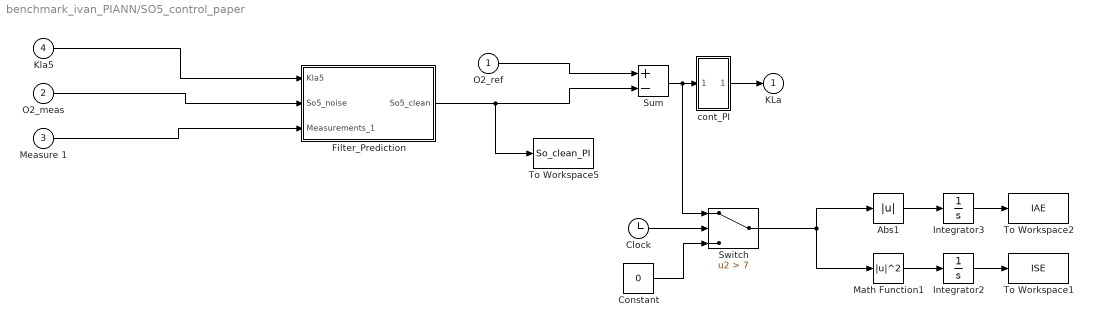
== system benchmark_ivan_PIANN/SO5_control_paper ==
  O2_ref : Inport
  O2_meas : Inport  Port=2
  Measure 1 : Inport  Port=3
  Kla5 : Inport  Port=4
  Abs1 : Abs  SaturateOnIntegerOverflow=off
  Clock : Clock
  Constant : Constant  Value=0
  Filter_Prediction : Subsystem
  Integrator2 : Integrator
  Integrator3 : Integrator
  Math Function1 : Math  Operator=magnitude^2  SignedPower=on
  Sum : Sum  Inputs=+-  InputSameDT=on  SaturateOnIntegerOverflow=on  OutDataTypeStr=Inherit: Same as first input
  Switch : Switch  Criteria=u2 > Threshold  Threshold=7  SaturateOnIntegerOverflow=off  InputSameDT=off
  To Workspace1 : ToWorkspace  VariableName=ISE  SampleTime=1/96
  To Workspace2 : ToWorkspace  VariableName=IAE  SampleTime=1/96
  To Workspace5 : ToWorkspace  VariableName=So_clean_PI  SampleTime=1/96
  cont_PI : Subsystem
  KLa : Outport  VectorParamsAs1DForOutWhenUnconnected=off
  wires:
  cont_PI/1(Out) -> KLa/1
  Sum/1 -> Switch/1, cont_PI/1(In)
  Math Function1/1 -> Integrator2/1
  Integrator2/1 -> To Workspace1/1
  Integrator3/1 -> To Workspace2/1
  Abs1/1 -> Integrator3/1
  Clock/1 -> Switch/2
  Switch/1 -> Abs1/1, Math Function1/1
  Constant/1 -> Switch/3
  Kla5/1 -> Filter_Prediction/1(Kla5)
  Measure 1/1 -> Filter_Prediction/3(Measurements_1)
  O2_ref/1 -> Sum/1
  Filter_Prediction/1(So5_clean) -> To Workspace5/1, Sum/2
  O2_meas/1 -> Filter_Prediction/2(So5_noise)

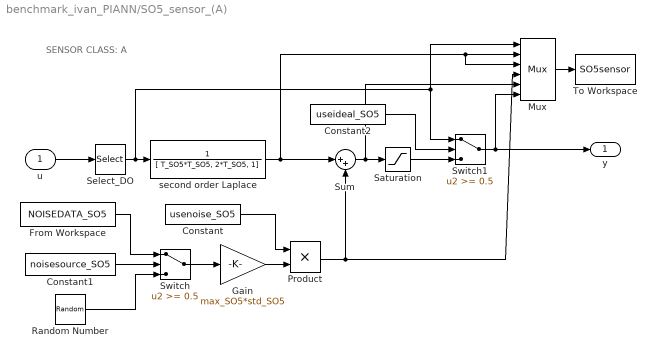
== system benchmark_ivan_PIANN/SO5_sensor_(A) ==
  note: SENSOR CLASS: A
  u : Inport
  Constant : Constant  Value=usenoise_SO5
  Constant1 : Constant  Value=noisesource_SO5
  Constant2 : Constant  Value=useideal_SO5
  From Workspace : FromWorkspace  VariableName=NOISEDATA_SO5  ZeroCross=off
  Gain : Gain  Gain=max_SO5*std_SO5  SaturateOnIntegerOverflow=on  OutDataTypeStr=Inherit: Same as input  ParamDataTypeStr=Inherit: Same as input
  Mux : Mux  Inputs=6
  Product : Product  InputSameDT=on  SaturateOnIntegerOverflow=on  OutDataTypeStr=Inherit: Same as first input
  Random Number : RandomNumber  Seed=noiseseed_SO5  SampleTime=1/10000
  Saturation : Saturate  UpperLimit=max_SO5  LowerLimit=min_SO5
  Select_DO : Selector  InputPortWidth=15  IndexOptions=Index vector (dialog)  Indices=[8]  OutputSizes=1
  Sum : Sum  Inputs=|++  InputSameDT=on  SaturateOnIntegerOverflow=on  OutDataTypeStr=Inherit: Same as first input
  Switch : Switch  Threshold=0.5  SaturateOnIntegerOverflow=off  InputSameDT=off
  Switch1 : Switch  Threshold=0.5  SaturateOnIntegerOverflow=off  InputSameDT=off
  To Workspace : ToWorkspace  VariableName=SO5sensor  SampleTime=-1
  second order Laplace : TransferFcn  Denominator=[ T_SO5*T_SO5, 2*T_SO5, 1]
  y : Outport  VectorParamsAs1DForOutWhenUnconnected=off
  wires:
  Mux/1 -> To Workspace/1
  Constant2/1 -> Switch1/2
  Switch1/1 -> Mux/6, y/1
  Saturation/1 -> Switch1/3
  Random Number/1 -> Switch/3
  Constant1/1 -> Switch/2
  From Workspace/1 -> Switch/1
  Constant/1 -> Product/1
  Switch/1 -> Gain/1
  Gain/1 -> Product/2
  Select_DO/1 -> Mux/1, Switch1/1, second order Laplace/1
  u/1 -> Select_DO/1
  Product/1 -> Mux/4, Sum/2
  second order Laplace/1 -> Mux/3, Mux/2, Sum/1
  Sum/1 -> Mux/5, Saturation/1

== system benchmark_ivan_PIANN/Settler_1D ==
  feed : Inport
  Qr : Inport  Port=2
  Qw : Inport  Port=3
  RAS underflow : Selector  InputPortWidth=113  IndexOptions=Index vector (dialog)  Indices=[1 2 3 4 5 6 7 8 9 10 11 12 13 14 15]  OutputSizes=1
  Settler_1D : S-Function  FunctionName=settler1dv4  Parameters=SETTLERINIT,SETTLERPAR,DIM,LAYER,MODELTYPE  SFunctionDeploymentMode=off  EnableBusSupport=off
  Store_feed : ToWorkspace  VariableName=feed  SampleTime=-1
  Store_settler : ToWorkspace  VariableName=settler  SampleTime=-1
  add Qr and Qw : Mux  Inputs=3
  output : Outport  VectorParamsAs1DForOutWhenUnconnected=off
  Settler : Outport  Port=2
  wires:
  add Qr and Qw/1 -> Settler_1D/1
  Qr/1 -> add Qr and Qw/2
  Qw/1 -> add Qr and Qw/3
  feed/1 -> add Qr and Qw/1, Store_feed/1
  RAS underflow/1 -> output/1
  Settler_1D/1 -> RAS underflow/1, Settler/1, Store_settler/1

== system benchmark_ivan_PIANN/Subsystem1 ==
  Add : Sum
  KLa mean : Constant  Value=So_mean
  KLa variations : FromWorkspace  VariableName=So_ref  SampleTime=-1  ZeroCross=off  OutputAfterFinalValue=Holding final value
  Select input : ManualSwitch
  To Workspace : ToWorkspace  VariableName=So5_sim  SampleTime=t_simulink
  To Workspace1 : ToWorkspace  VariableName=So5_sim_p  SampleTime=t_simulink
  Transfer Fcn : TransferFcn  Commented=on  Denominator=[t_init 1]
  Transfer Fcn1 : TransferFcn  Commented=on  Denominator=[t_init 1]
  Transport Delay : TransportDelay  DelayTime=10/(60*24)
  So5_ref : Outport  VectorParamsAs1DForOutWhenUnconnected=off
  wires:
  Transport Delay/1 -> To Workspace1/1
  KLa variations/1 -> Select input/1, Transfer Fcn1/1
  Transfer Fcn1/1 -> Select input/2
  Select input/1 -> Add/1
  Add/1 -> To Workspace/1, Transport Delay/1, So5_ref/1
  KLa mean/1 -> Add/2

== system benchmark_ivan_PIANN/Subsystem2 ==
  Add : Sum
  KLa mean : Constant  Value=Sno_mean
  KLa variations : FromWorkspace  VariableName=Sno_ref  SampleTime=-1  ZeroCross=off  OutputAfterFinalValue=Holding final value
  Select input : ManualSwitch
  To Workspace : ToWorkspace  VariableName=Sno2_sim  SampleTime=t_simulink
  To Workspace1 : ToWorkspace  VariableName=Sno2_sim_p  SampleTime=t_simulink
  Transfer Fcn : TransferFcn  Commented=on  Denominator=[t_init 1]
  Transfer Fcn1 : TransferFcn  Commented=on  Denominator=[t_init 1]
  Transport Delay : TransportDelay  DelayTime=10/(60*24)
  Sno2_ref : Outport  VectorParamsAs1DForOutWhenUnconnected=off
  wires:
  Transport Delay/1 -> To Workspace1/1
  KLa variations/1 -> Select input/1, Transfer Fcn1/1
  Transfer Fcn1/1 -> Select input/2
  Select input/1 -> Add/1
  Add/1 -> To Workspace/1, Transport Delay/1, Sno2_ref/1
  KLa mean/1 -> Add/2

== system benchmark_ivan_PIANN/Bioreactor_1/Carboncombiner ==
  C_flow : Inport
  Input : Inport  Port=2
  Carboncombiner : S-Function  FunctionName=carboncombiner  Parameters=CARBONSOURCECONC  SFunctionDeploymentMode=off  EnableBusSupport=off
  Mux : Mux  Inputs=2
  Output : Outport  VectorParamsAs1DForOutWhenUnconnected=off
  wires:
  C_flow/1 -> Mux/1
  Mux/1 -> Carboncombiner/1
  Carboncombiner/1 -> Output/1
  Input/1 -> Mux/2

== system benchmark_ivan_PIANN/Bioreactor_2/Carboncombiner ==
  C_flow : Inport
  Input : Inport  Port=2
  Carboncombiner : S-Function  FunctionName=carboncombiner  Parameters=CARBONSOURCECONC  SFunctionDeploymentMode=off  EnableBusSupport=off
  Mux : Mux  Inputs=2
  Output : Outport  VectorParamsAs1DForOutWhenUnconnected=off
  wires:
  Input/1 -> Mux/2
  Carboncombiner/1 -> Output/1
  Mux/1 -> Carboncombiner/1
  C_flow/1 -> Mux/1

== system benchmark_ivan_PIANN/Bioreactor_3/Carboncombiner ==
  C_flow : Inport
  Input : Inport  Port=2
  Carboncombiner : S-Function  FunctionName=carboncombiner  Parameters=CARBONSOURCECONC  SFunctionDeploymentMode=off  EnableBusSupport=off
  Mux : Mux  Inputs=2
  Output : Outport  VectorParamsAs1DForOutWhenUnconnected=off
  wires:
  Input/1 -> Mux/2
  Carboncombiner/1 -> Output/1
  Mux/1 -> Carboncombiner/1
  C_flow/1 -> Mux/1

== system benchmark_ivan_PIANN/Bioreactor_4/Carboncombiner ==
  C_flow : Inport
  Input : Inport  Port=2
  Carboncombiner : S-Function  FunctionName=carboncombiner  Parameters=CARBONSOURCECONC  SFunctionDeploymentMode=off  EnableBusSupport=off
  Mux : Mux  Inputs=2
  Output : Outport  VectorParamsAs1DForOutWhenUnconnected=off
  wires:
  Input/1 -> Mux/2
  Carboncombiner/1 -> Output/1
  Mux/1 -> Carboncombiner/1
  C_flow/1 -> Mux/1

== system benchmark_ivan_PIANN/Bioreactor_5/Carboncombiner ==
  C_flow : Inport
  Input : Inport  Port=2
  Carboncombiner : S-Function  FunctionName=carboncombiner  Parameters=CARBONSOURCECONC  SFunctionDeploymentMode=off  EnableBusSupport=off
  Mux : Mux  Inputs=2
  Output : Outport  VectorParamsAs1DForOutWhenUnconnected=off
  wires:
  Input/1 -> Mux/2
  Carboncombiner/1 -> Output/1
  Mux/1 -> Carboncombiner/1
  C_flow/1 -> Mux/1

== system benchmark_ivan_PIANN/Direct Prediction 2 LSTM SO1/Data Preprocesing Direct ==
  u_n : Inport
  Math Function : Math  Operator=transpose  SignedPower=on
  Normalizer1 : Subsystem
  Reshape : Reshape  OutputDimensionality=Row vector (2-D)
  Out1 : Outport  VectorParamsAs1DForOutWhenUnconnected=off
  wires:
  u_n/1 -> Normalizer1/1(Data Input)
  Math Function/1 -> Reshape/1
  Normalizer1/1(Data Normalized) -> Math Function/1
  Reshape/1 -> Out1/1

== system benchmark_ivan_PIANN/Direct Prediction 2 LSTM SO1/Data Preprocessing Direct1 ==
  y_n : Inport
  Denormalization Values : MATLAB Function  TreatAsAtomicUnit=on
  Out1 : Outport  VectorParamsAs1DForOutWhenUnconnected=off
  wires:
  Denormalization Values/1(data_dir) -> Out1/1
  y_n/1 -> Denormalization Values/1(data_input)

== system benchmark_ivan_PIANN/Direct Prediction 2 LSTM SO1/Direct ANN1 ==
  x_norm : Inport
  Predict RNN Ntot Keras : MATLAB Function  TreatAsAtomicUnit=on
  y_n : Outport  VectorParamsAs1DForOutWhenUnconnected=off
  wires:
  x_norm/1 -> Predict RNN Ntot Keras/1(data_in)
  Predict RNN Ntot Keras/1(prediction) -> y_n/1

== system benchmark_ivan_PIANN/Direct Prediction 2 LSTM SO1/IAE_ISE ==
  In1 : Inport
  Abs1 : Abs  SaturateOnIntegerOverflow=off
  Clock1 : Clock
  Constant : Constant  Value=0
  Integrator2 : Integrator
  Integrator3 : Integrator
  Math Function1 : Math  Operator=magnitude^2  SignedPower=on
  Switch : Switch  Criteria=u2 > Threshold  Threshold=7  SaturateOnIntegerOverflow=off  InputSameDT=off
  To Workspace1 : ToWorkspace  VariableName=ISE_So5  SampleTime=-1
  To Workspace2 : ToWorkspace  VariableName=IAE_So5  SampleTime=-1
  wires:
  Clock1/1 -> Switch/2
  Abs1/1 -> Integrator3/1
  In1/1 -> Switch/1
  Constant/1 -> Switch/3
  Integrator3/1 -> To Workspace2/1
  Integrator2/1 -> To Workspace1/1
  Switch/1 -> Math Function1/1, Abs1/1
  Math Function1/1 -> Integrator2/1

== system benchmark_ivan_PIANN/Direct Prediction 2 LSTM SO1/Sliding Window ==
  So5sim : Inport
  So5out : Inport  Port=2
  errorSo5 : Inport  Port=3
  kla : Inport  Port=4
  Matrix Concatenate : Concatenate  NumInputs=4  Mode=Multidimensional array  ConcatenateDimension=2
  Sliding Window Buffer So1 : Subsystem  Commented=on
  Sliding Window Buffer So2 : Subsystem  Commented=on
  Sliding Window Buffer So3 : Subsystem  Commented=on
  Sliding Window Buffer So4 : Subsystem  Commented=on
  Zero-Order Hold{,1..3} (4 alike) : ZeroOrderHold  SampleTime=-1
  Out1 : Outport
  wires:
  Zero-Order Hold3/1 -> Matrix Concatenate/4
  Zero-Order Hold2/1 -> Matrix Concatenate/3
  Zero-Order Hold1/1 -> Matrix Concatenate/2
  Zero-Order Hold/1 -> Matrix Concatenate/1
  kla/1 -> Zero-Order Hold3/1
  errorSo5/1 -> Zero-Order Hold2/1
  So5out/1 -> Zero-Order Hold1/1
  So5sim/1 -> Zero-Order Hold/1
  Matrix Concatenate/1 -> Out1/1

== system benchmark_ivan_PIANN/Direct Prediction LSTM3/Data Preprocesing Direct ==
  u_n : Inport
  Math Function : Math  Operator=transpose  SignedPower=on
  Normalizer1 : Subsystem
  Reshape : Reshape  OutputDimensionality=Row vector (2-D)
  Out1 : Outport  VectorParamsAs1DForOutWhenUnconnected=off
  wires:
  Reshape/1 -> Out1/1
  Normalizer1/1(Data Normalized) -> Math Function/1
  Math Function/1 -> Reshape/1
  u_n/1 -> Normalizer1/1(Data Input)

== system benchmark_ivan_PIANN/Direct Prediction LSTM3/Data Preprocessing Direct1 ==
  y_n : Inport
  Denormalization Values : MATLAB Function  TreatAsAtomicUnit=on
  Out1 : Outport  VectorParamsAs1DForOutWhenUnconnected=off
  wires:
  y_n/1 -> Denormalization Values/1(data_input)
  Denormalization Values/1(data_dir) -> Out1/1

== system benchmark_ivan_PIANN/Direct Prediction LSTM3/Direct ANN ==
  x_norm : Inport
  Predict RNN Ntot Keras : MATLAB Function  TreatAsAtomicUnit=on
  y_n : Outport  VectorParamsAs1DForOutWhenUnconnected=off
  wires:
  Predict RNN Ntot Keras/1(prediction) -> y_n/1
  x_norm/1 -> Predict RNN Ntot Keras/1(data_in)

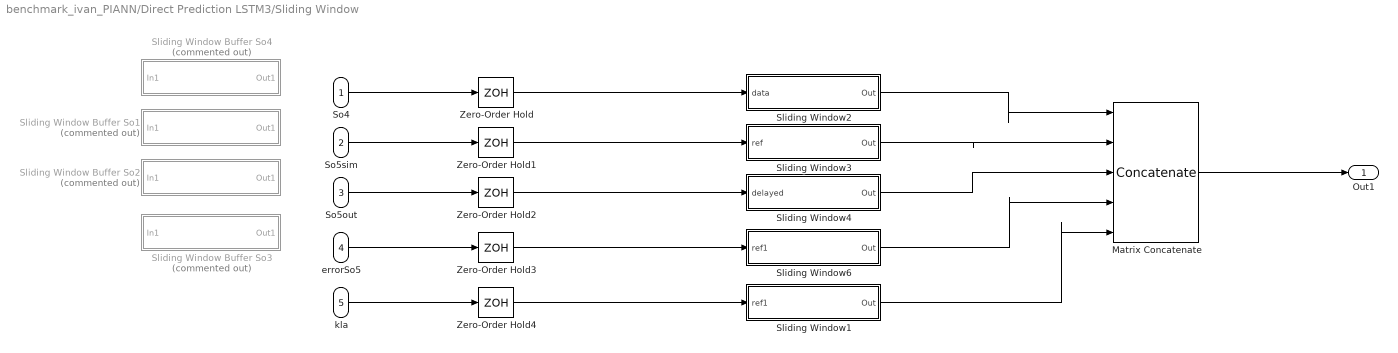
== system benchmark_ivan_PIANN/Direct Prediction LSTM3/Sliding Window ==
  So4 : Inport
  So5sim : Inport  Port=2
  So5out : Inport  Port=3
  errorSo5 : Inport  Port=4
  kla : Inport  Port=5
  Matrix Concatenate : Concatenate  NumInputs=5  Mode=Multidimensional array  ConcatenateDimension=2
  Sliding Window Buffer So1 : Subsystem  Commented=on
  Sliding Window Buffer So2 : Subsystem  Commented=on
  Sliding Window Buffer So3 : Subsystem  Commented=on
  Sliding Window Buffer So4 : Subsystem  Commented=on
  Sliding Window1 : Subsystem
  Sliding Window2 : Subsystem
  Sliding Window3 : Subsystem
  Sliding Window4 : Subsystem
  Sliding Window6 : Subsystem
  Zero-Order Hold{,1..4} (5 alike) : ZeroOrderHold  SampleTime=-1
  Out1 : Outport
  wires:
  Sliding Window2/1(Out) -> Matrix Concatenate/1
  Sliding Window3/1(Out) -> Matrix Concatenate/2
  Sliding Window4/1(Out) -> Matrix Concatenate/3
  Sliding Window6/1(Out) -> Matrix Concatenate/4
  Matrix Concatenate/1 -> Out1/1
  So4/1 -> Zero-Order Hold/1
  So5sim/1 -> Zero-Order Hold1/1
  So5out/1 -> Zero-Order Hold2/1
  errorSo5/1 -> Zero-Order Hold3/1
  kla/1 -> Zero-Order Hold4/1
  Sliding Window1/1(Out) -> Matrix Concatenate/5
  Zero-Order Hold/1 -> Sliding Window2/1(data)
  Zero-Order Hold1/1 -> Sliding Window3/1(ref)
  Zero-Order Hold2/1 -> Sliding Window4/1(delayed)
  Zero-Order Hold3/1 -> Sliding Window6/1(ref1)
  Zero-Order Hold4/1 -> Sliding Window1/1(ref1)

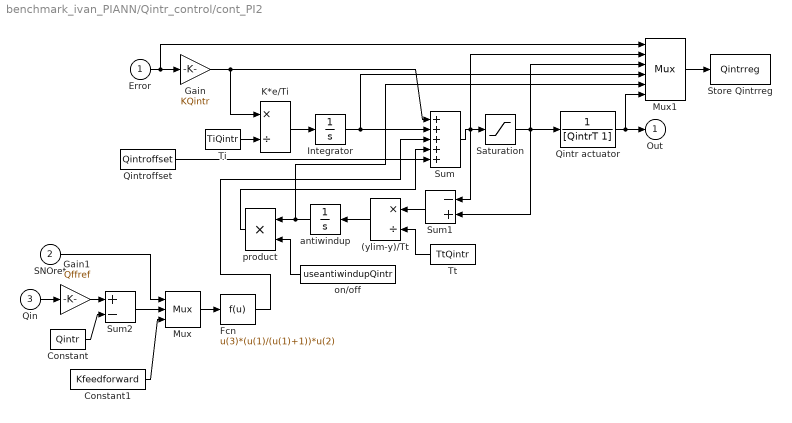
== system benchmark_ivan_PIANN/Qintr_control/cont_PI2 ==
  Error : Inport
  SNOref : Inport  Port=2
  Qin : Inport  Port=3
  (ylim-y)/Tt : Product  Inputs=*/  InputSameDT=on  SaturateOnIntegerOverflow=on  OutDataTypeStr=Inherit: Same as first input
  Constant : Constant  Value=Qintr
  Constant1 : Constant  Value=Kfeedforward
  Fcn : Fcn  Expr=u(3)*(u(1)/(u(1)+1))*u(2)
  Gain : Gain  Gain=KQintr  SaturateOnIntegerOverflow=on  OutDataTypeStr=Inherit: Same as input  ParamDataTypeStr=Inherit: Same as input
  Gain1 : Gain  Gain=Qffref  SaturateOnIntegerOverflow=on  OutDataTypeStr=Inherit: Same as input  ParamDataTypeStr=Inherit: Same as input
  Integrator : Integrator  InitialCondition=Qintrintstate
  K*e/Ti : Product  Inputs=*/  InputSameDT=on  SaturateOnIntegerOverflow=on  OutDataTypeStr=Inherit: Same as first input
  Mux : Mux  Inputs=3
  Mux1 : Mux  Inputs=6
  Qintr actuator : TransferFcn  Denominator=[QintrT 1]
  Qintroffset : Constant  Value=Qintroffset
  Saturation : Saturate  UpperLimit=Qintr_max  LowerLimit=0
  Store Qintrreg : ToWorkspace  VariableName=Qintrreg  SampleTime=-1
  Sum : Sum  Inputs=+++++  InputSameDT=on  SaturateOnIntegerOverflow=on  OutDataTypeStr=Inherit: Same as first input
  Sum1 : Sum  Inputs=-+  InputSameDT=on  SaturateOnIntegerOverflow=on  OutDataTypeStr=Inherit: Same as first input
  Sum2 : Sum  Inputs=+-  InputSameDT=on  SaturateOnIntegerOverflow=on  OutDataTypeStr=Inherit: Same as first input
  Ti : Constant  Value=TiQintr
  Tt : Constant  Value=TtQintr
  antiwindup : Integrator  InitialCondition=Qintrawstate
  on/off : Constant  Value=useantiwindupQintr
  product : Product  Inputs=**  InputSameDT=on  SaturateOnIntegerOverflow=on  OutDataTypeStr=Inherit: Same as first input
  Out : Outport  VectorParamsAs1DForOutWhenUnconnected=off
  wires:
  Sum2/1 -> Mux/2
  Constant1/1 -> Mux/3
  on/off/1 -> product/2
  Error/1 -> Mux1/1, Gain/1
  Mux1/1 -> Store Qintrreg/1
  Saturation/1 -> Sum1/2, Qintr actuator/1, Mux1/3
  Sum/1 -> Mux1/2, Sum1/1, Saturation/1
  (ylim-y)/Tt/1 -> antiwindup/1
  Tt/1 -> (ylim-y)/Tt/2
  Sum1/1 -> (ylim-y)/Tt/1
  Gain/1 -> Sum/1, K*e/Ti/1
  Ti/1 -> K*e/Ti/2
  K*e/Ti/1 -> Integrator/1
  product/1 -> Sum/4
  SNOref/1 -> Mux/1
  Mux/1 -> Fcn/1
  Fcn/1 -> Sum/3
  Integrator/1 -> Sum/2, Mux1/4
  antiwindup/1 -> product/1, Mux1/5
  Constant/1 -> Sum2/2
  Qin/1 -> Gain1/1
  Gain1/1 -> Sum2/1
  Qintroffset/1 -> Sum/5
  Qintr actuator/1 -> Out/1, Mux1/6

== system benchmark_ivan_PIANN/SO5_control1/Filter_Prediction1 ==
  Kla5 : Inport
  So5_noise : Inport  Port=2
  Measurements : Inport  Port=3
  DAE_MLP2 : Subsystem
  Direct Prediction LSTM4 : Subsystem
  SNH4_sensor_(B0) : Subsystem
  SNO4_sensor_(B0) : Subsystem
  SO4_sensor_(A) : Subsystem
  To Workspace5 : ToWorkspace  Commented=on  VariableName=clean_data  SampleTime=1/96
      settings: Save2DSignal=2-D array (concatenate along first dimension)
  So5_clean : Outport
  wires:
  SO4_sensor_(A)/1(y) -> DAE_MLP2/1(So4)
  SNO4_sensor_(B0)/1(y) -> DAE_MLP2/2(Sno4)
  SNH4_sensor_(B0)/1(y) -> DAE_MLP2/3(Snh4)
  Kla5/1 -> Direct Prediction LSTM4/1(kla1)
  Measurements/1 -> SO4_sensor_(A)/1(u), SNO4_sensor_(B0)/1(u), SNH4_sensor_(B0)/1(u)
  DAE_MLP2/1(Output) -> Direct Prediction LSTM4/2(meas1), To Workspace5/1
  So5_noise/1 -> DAE_MLP2/4("So5_noise ")
  Direct Prediction LSTM4/1(y_n) -> So5_clean/1
